simulink model "empc_stirling_sim"  (Simulink 8.8)
settings: Solver=ode45  StartTime=0.0  StopTime=Tsim  RelTol=1e-3  EnableMultiTasking=on
values from neighbouring files (symbols this model uses):
  a = [-0.1832;558;118.45;9.6154e+03;     1.3712;5.1011e+03;641;426;6557;7.34;4484;0.016]    [script.m]
  k = 1    [script.m]
  Ts = 1e-4    (= 0.0001)    [script.m]
  x5d = 50    [script.m]
undefined symbols (not defined in the file or in its folder): empc_control, rsSVM, ud, wienerModel, xd
settings Model: Creator=TIEUPHI  LastModifiedBy=trinhvv-admin
settings DataIOCC: SaveFormat=StructureWithTime  SignalLoggingSaveFormat=Dataset
settings DebuggingCC: UnderspecifiedInitializationDetection=Simplified  MergeDetectMultiDrivingBlocksExec=error  AllowSymbolicDim=off  StateNameClashWarn=none
settings HardwareCC: ProdBitPerPointer=64  ProdLargestAtomicFloat=Float  ProdIntDivRoundTo=Zero  ProdEndianess=LittleEndian  ProdHWDeviceType=Specified
settings GRTTargetCC: GeneratePreprocessorConditionals=Use local settings  CombineOutputUpdateFcns=on  GRTInterface=off

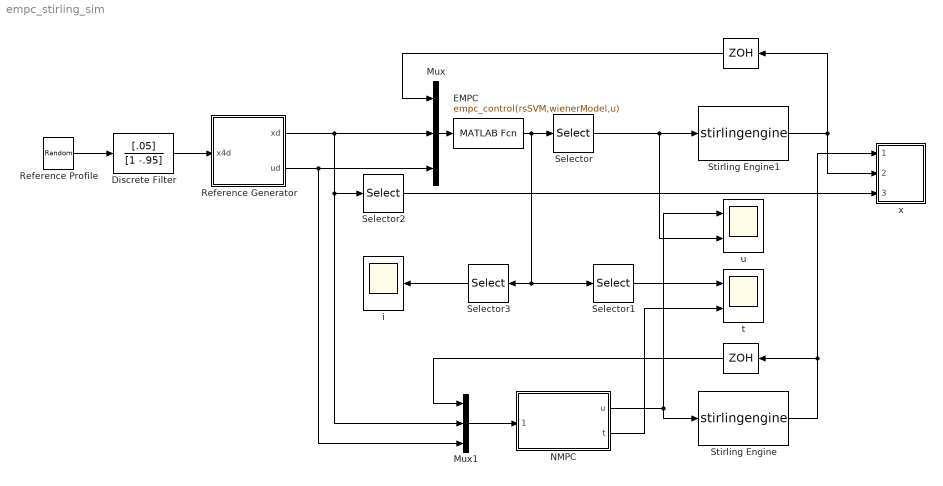
== system empc_stirling_sim ==
  "  " : ZeroOrderHold  SampleTime=Ts
  "                          " : ZeroOrderHold  SampleTime=Ts
  Discrete Filter : DiscreteFilter  Numerator=[.05]  Denominator=[1 -.95]  InitialStates=10.08*20  SampleTime=1e-3
  EMPC : MATLABFcn  MATLABFcn=empc_control(rsSVM,wienerModel,u)  OutputDimensions=3
  Mux : Mux  Inputs=3
  Mux1 : Mux  Inputs=3
  NMPC : Subsystem
  Reference Generator : Subsystem
      mask init:
      | load ref_gen;
  Reference Profile : UniformRandomNumber  Minimum=7  Maximum=13  Seed=3213456789  SampleTime=.5
  Selector : Selector  InputPortWidth=3  IndexOptions=Index vector (dialog)  Indices=1  OutputSizes=1
  Selector1 : Selector  InputPortWidth=3  IndexOptions=Index vector (dialog)  Indices=3  OutputSizes=1
  Selector2 : Selector  InputPortWidth=4  IndexOptions=Index vector (dialog)  Indices=4  OutputSizes=1
  Selector3 : Selector  InputPortWidth=3  IndexOptions=Index vector (dialog)  Indices=2  OutputSizes=1
  Stirling Engine : S-Function  InitFcn=try, set_param(gcb,'FunctionName','stirlingengine'), end  FunctionName=stirlingengine  Parameters=a,k,x5d  SFunctionModules=stirlingengine_wrapper  WizardData=DataTag0  SFunctionDeploymentMode=off  EnableBusSupport=off  mask(S-Function Builder){}
      mask help: Simulink:masks:SFunctionBuilder_MD
      mask init:
      | val = [[.9  0.75 0.75 1 1 .9 .9 1]',[1 1 0.75 0.75 .9 .9 1 .9]'];try , sys = get_param(gcb,'SfunBuilderFcnName');if isempty(sys), sys = get_param(gcb,'FunctionName'); end,catch, sys = get_param(gcb,'FunctionName'); end
      settings: CopyFcn=set_param(gcbh,'LinkStatus','none')  PreSaveFcn=try, set_param(gcb,'FunctionName','stirlingengine'), end  OpenFcn=sfunctionwizard(gcbh)
      mask Display: plot(val(:,1),val(:,2)),disp(sys), port_label('input',1,'u'), port_label('output',1,'y')
  Stirling Engine1 : S-Function  InitFcn=try, set_param(gcb,'FunctionName','stirlingengine'), end  FunctionName=stirlingengine  Parameters=a,k,x5d  SFunctionModules=stirlingengine_wrapper  WizardData=DataTag1  SFunctionDeploymentMode=off  EnableBusSupport=off  mask(S-Function Builder){}
      mask help: Simulink:masks:SFunctionBuilder_MD
      mask init: same as empc_stirling_sim/Stirling Engine
      settings: CopyFcn=set_param(gcbh,'LinkStatus','none')  PreSaveFcn=try, set_param(gcb,'FunctionName','stirlingengine'), end  OpenFcn=sfunctionwizard(gcbh)
      mask Display: plot(val(:,1),val(:,2)),disp(sys), port_label('input',1,'u'), port_label('output',1,'y')
  i : Scope
  t : Scope  NumInputPorts=2
  u : Scope  NumInputPorts=2
  x : Subsystem
  wires:
  Mux/1 -> EMPC/1
  Stirling Engine1/1 -> "                          "/1, x/2("   ")
  Reference Profile/1 -> Discrete Filter/1
  "                          "/1 -> Mux/1
  EMPC/1 -> Selector/1, Selector1/1, Selector3/1
  Selector1/1 -> t/1
  Mux1/1 -> NMPC/1(" ")
  Stirling Engine/1 -> x/1(" "), "  "/1
  "  "/1 -> Mux1/1
  NMPC/1(u) -> Stirling Engine/1, u/1
  Discrete Filter/1 -> Reference Generator/1(x4d)
  Reference Generator/1(xd) -> Mux/2, Selector2/1, Mux1/2
  Selector2/1 -> x/3("          ")
  Reference Generator/2(ud) -> Mux/3, Mux1/3
  Selector3/1 -> i/1
  NMPC/2(t) -> t/2
  Selector/1 -> u/2, Stirling Engine1/1

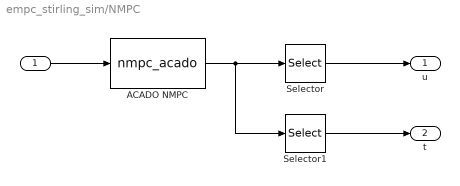
== system empc_stirling_sim/NMPC ==
  " " : Inport
  ACADO NMPC : MATLABFcn  MATLABFcn=nmpc_acado  OutputDimensions=2  OutputSignalType=real  SampleTime=Ts
  Selector : Selector  IndexOptions=Index vector (dialog)  Indices=1  OutputSizes=1
  Selector1 : Selector  IndexOptions=Index vector (dialog)  Indices=2  OutputSizes=1
  u : Outport
  t : Outport  Port=2
  wires:
  " "/1 -> ACADO NMPC/1
  ACADO NMPC/1 -> Selector1/1, Selector/1
  Selector/1 -> u/1
  Selector1/1 -> t/1

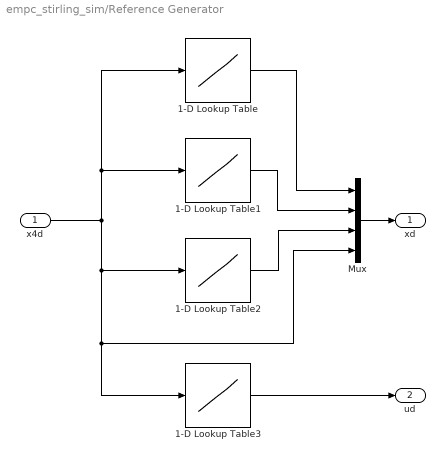
== system empc_stirling_sim/Reference Generator ==
  x4d : Inport
  1-D Lookup Table : Lookup_n-D  NumberOfTableDimensions=1  BreakpointsForDimension1=xd(:,4)  Table=xd(:,1)  RndMeth=Simplest  InputSameDT=on
  1-D Lookup Table1 : Lookup_n-D  NumberOfTableDimensions=1  BreakpointsForDimension1=xd(:,4)  Table=xd(:,2)  RndMeth=Simplest  InputSameDT=on
  1-D Lookup Table2 : Lookup_n-D  NumberOfTableDimensions=1  BreakpointsForDimension1=xd(:,4)  Table=xd(:,3)  RndMeth=Simplest  InputSameDT=on
  1-D Lookup Table3 : Lookup_n-D  NumberOfTableDimensions=1  BreakpointsForDimension1=xd(:,4)  Table=ud  RndMeth=Simplest  InputSameDT=on
  Mux : Mux
  xd : Outport
  ud : Outport  Port=2
  wires:
  x4d/1 -> Mux/4, 1-D Lookup Table3/1, 1-D Lookup Table2/1, 1-D Lookup Table1/1, 1-D Lookup Table/1
  Mux/1 -> xd/1
  1-D Lookup Table/1 -> Mux/1
  1-D Lookup Table1/1 -> Mux/2
  1-D Lookup Table2/1 -> Mux/3
  1-D Lookup Table3/1 -> ud/1

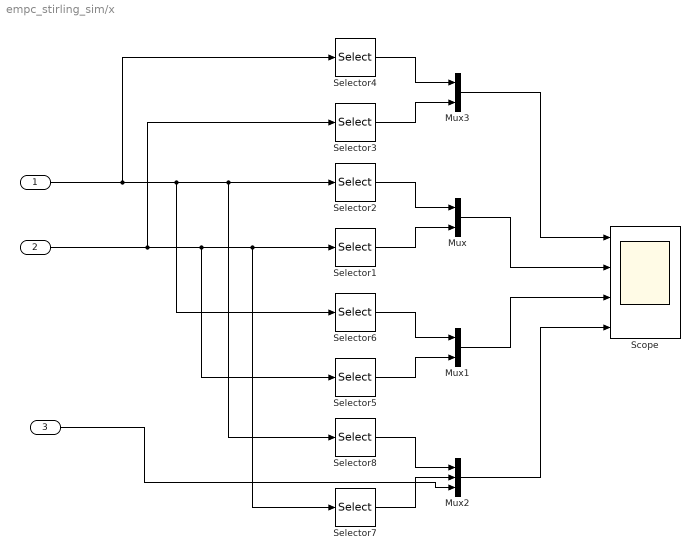
== system empc_stirling_sim/x ==
  " " : Inport
  "   " : Inport  Port=2
  "          " : Inport  Port=3
  Mux : Mux  Inputs=2
  Mux1 : Mux  Inputs=2
  Mux2 : Mux  Inputs=3
  Mux3 : Mux  Inputs=2
  Scope : Scope  NumInputPorts=4
  Selector1 : Selector  InputPortWidth=4  IndexOptions=Index vector (dialog)  Indices=2  OutputSizes=1
  Selector2 : Selector  InputPortWidth=4  IndexOptions=Index vector (dialog)  Indices=2  OutputSizes=1
  Selector3 : Selector  InputPortWidth=4  IndexOptions=Index vector (dialog)  Indices=1  OutputSizes=1
  Selector4 : Selector  InputPortWidth=4  IndexOptions=Index vector (dialog)  Indices=1  OutputSizes=1
  Selector5 : Selector  InputPortWidth=4  IndexOptions=Index vector (dialog)  Indices=3  OutputSizes=1
  Selector6 : Selector  InputPortWidth=4  IndexOptions=Index vector (dialog)  Indices=3  OutputSizes=1
  Selector7 : Selector  InputPortWidth=4  IndexOptions=Index vector (dialog)  Indices=4  OutputSizes=1
  Selector8 : Selector  InputPortWidth=4  IndexOptions=Index vector (dialog)  Indices=4  OutputSizes=1
  wires:
  Selector1/1 -> Mux/2
  Selector2/1 -> Mux/1
  "   "/1 -> Selector3/1, Selector5/1, Selector7/1, Selector1/1
  " "/1 -> Selector6/1, Selector8/1, Selector2/1, Selector4/1
  Selector5/1 -> Mux1/2
  Selector6/1 -> Mux1/1
  Selector7/1 -> Mux2/2
  Mux2/1 -> Scope/4
  Selector3/1 -> Mux3/2
  Selector4/1 -> Mux3/1
  Mux1/1 -> Scope/3
  Mux/1 -> Scope/2
  Mux3/1 -> Scope/1
  Selector8/1 -> Mux2/1
  "          "/1 -> Mux2/3
